simulink model "rf_satlink"  (Simulink 6.0)
settings: Solver=ode45  StartTime=0.0  StopTime=Inf  RelTol=1e-3
undefined symbols (not defined in the file or in its folder): Fs, magnitude, slcm
libraries: commrflib2 x7, commsink2 x5, dsparch4 x4, commfilt2 x2, commdigbbndam2 x2, dspsrcs4 x2, simulink x1, dspsnks4 x1, commrandsrc2 x1
CloseFcn:
  | clear satlinkSigsOut method model_type
settings Model: Creator=mclune  LastModifiedBy=arodrigu  ExtModeAutoUpdateStatusClock=off  BufferReuse=off
settings DataIOCC: SaveOutput=off  SaveTime=off  SignalLoggingName=satlinkSigsOut
settings OptimizationCC: OptimizeBlockIOStorage=off  BufferReuse=off  ExpressionFolding=off  LocalBlockOutputs=off
settings DebuggingCC: CheckExecutionContextPreStartOutputMsg=on  CheckExecutionContextRuntimeOutputMsg=on  SolverPrmCheckMsg=none  InheritedTsInSrcMsg=none
settings HardwareCC: TargetUnknown=on
settings ModelReferenceCC: UpdateModelReferenceTargets=IfOutOfDate

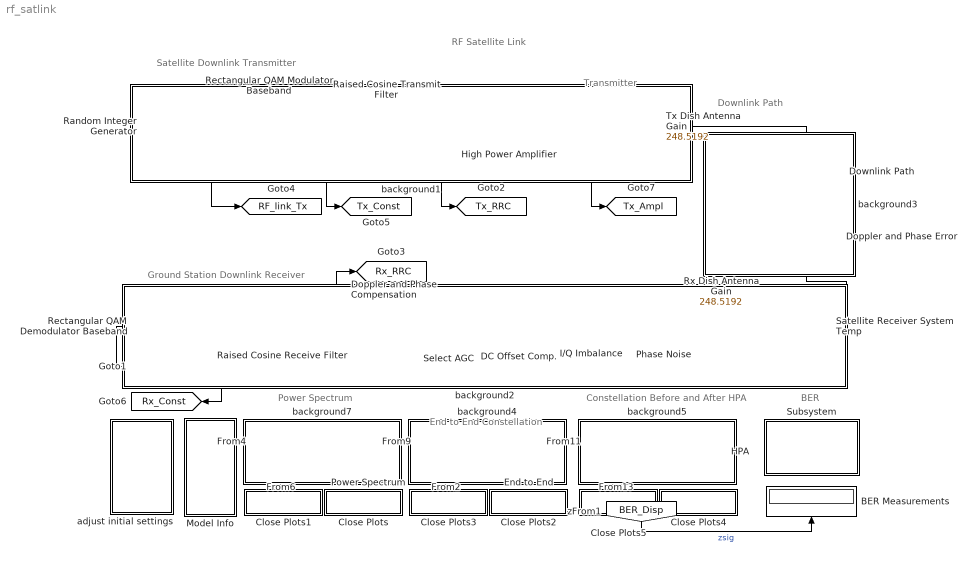
== system rf_satlink ==
  note: RF Satellite Link
  note: Constellation Before and After HPA
  note: Power Spectrum
  note: Downlink Path
  note: Satellite Downlink Transmitter
  note: Transmitter
  note: Ground Station Downlink Receiver
  note: End to End Constellation
  note: BER
  BER Measurements : Display
      settings: Orientation=up
  Close Plots : Subsystem  PropExecContextAcrossSSBoundary=on
      settings: OpenFcn=|
      | sdspfscope2([],[],[],'ScopeUpdate',[gcs '/Power Spectrum/Tx and Rx Spectrum'],'CloseFig');
      | set_param([gcs '/Power Spectrum/Tx and Rx Spectrum'],'OpenScopeAtSimStart','off');
      mask Display: disp('Close Scopes');
  Close Plots1 : Subsystem  PropExecContextAcrossSSBoundary=on
      settings: OpenFcn=|
      | sdspfscope2([],[],[],'ScopeUpdate',[gcs '/Power Spectrum/Tx and Rx Spectrum'],'OpenFig');
      | set_param([gcs '/Power Spectrum/Tx and Rx Spectrum'],'OpenScopeAtSimStart','on');
      mask Display: disp('Open Scopes');
  Close Plots2 : Subsystem  PropExecContextAcrossSSBoundary=on
      settings: OpenFcn=|
      | sdspfscope2([],[],[],'ScopeUpdate',[gcs '/End to End/Transmit Constellation'],'CloseFig');
      |    sdspfscope2([],[],[],'ScopeUpdate',[gcs '/End to End/Received Constellation'],'CloseFig');
      |  set_param([gcs '/End to End/Transmit Constellation'],'OpenScopeAtSimStart','off');
      |    set_param([gcs '/End to End/Received Constellation'],'OpenScopeAtSimStart','off');
      mask Display: disp('Close Scopes');
  Close Plots3 : Subsystem  PropExecContextAcrossSSBoundary=on
      settings: OpenFcn=|
      | sdspfscope2([],[],[],'ScopeUpdate',[gcs '/End to End/Transmit Constellation'],'OpenFig');
      |     sdspfscope2([],[],[],'ScopeUpdate',[gcs '/End to End/Received Constellation'],'OpenFig');
      |   set_param([gcs '/End to End/Transmit Constellation'],'OpenScopeAtSimStart','on');
      |     set_param([gcs '/End to End/Received Constellation'],'OpenScopeAtSimStart','on');
      mask Display: disp('Open Scopes');
  Close Plots4 : Subsystem  PropExecContextAcrossSSBoundary=on
      settings: OpenFcn=|
      | sdspfscope2([],[],[],'ScopeUpdate',[gcs '/HPA/Transmit RRC filtered signal'],'CloseFig');
      |   set_param([gcs '/HPA/Transmit RRC filtered signal'],'OpenScopeAtSimStart','off');
      |     sdspfscope2([],[],[],'ScopeUpdate',[gcs '/HPA/RRC signal after HPA'],'CloseFig');
      |   set_param([gcs '/HPA/RRC signal after HPA'],'OpenScopeAtSimStart','off');
      mask Display: disp('Close Scopes');
  Close Plots5 : Subsystem  PropExecContextAcrossSSBoundary=on
      settings: OpenFcn=|
      | sdspfscope2([],[],[],'ScopeUpdate',[gcs '/HPA/Transmit RRC filtered signal'],'OpenFig');
      | set_param([gcs '/HPA/Transmit RRC filtered signal'],'OpenScopeAtSimStart','on');
      |   sdspfscope2([],[],[],'ScopeUpdate',[gcs '/HPA/RRC signal after HPA'],'OpenFig');
      | set_param([gcs '/HPA/RRC signal after HPA'],'OpenScopeAtSimStart','on');
      mask Display: disp('Open Scopes');
  DC Offset Comp. : Subsystem  Orientation=left  BlockChoice=Magnitude Only  PropExecContextAcrossSSBoundary=on
      mask Display: disp('DC\nRemoval')
  Doppler and Phase Error : commrflib2/Phase// Frequency Offset  Orientation=down  freqOffset=0  phaseOffset=0
  Doppler and Phase Compensation : commrflib2/Phase// Frequency Offset  Orientation=left  freqOffset=0  phaseOffset=0
  Downlink Path : commrflib2/Free Space Path Loss  Orientation=down  mode=Distance and Frequency  dB=180  d=35600  fc=8000
  End to End : Subsystem  TreatAsAtomicUnit=on  PropExecContextAcrossSSBoundary=on
      mask Display: disp('End-End\nScatter\nPlot')
  HPA : Subsystem  TreatAsAtomicUnit=on  PropExecContextAcrossSSBoundary=on
      mask Display: disp('HPA\nScatter\nPlot')
  High Power Amplifier : commrflib2/Memoryless Nonlinearity  model_select=Saleh model  linGaindB=16  GindB=-21.5957  iip3=30  am2pm=1  amam=[2.1587 1.1517]  ampm=[4.0330 9.1040]  x=[8.1081 1.5413 6.5202 -0.0718]  y=[4.6645 2.0965 10.88 -0.003]  p=0.3  GoutdB=32.9118  vsat=100
  I/Q Imbalance : commrflib2/I//Q Imbalance  Orientation=left  ampImbal=0  phsImbal=0  Idc=0  Qdc=0
  Model Info : Subsystem  LoadFcn=slcm LoadBlock;  InitFcn=slcm('UpdateAllCMBlocksInThisModelInit')  PropExecContextAcrossSSBoundary=on  mask(CMBlock){InitialSaveTempField=, InitialBlockCM=None, BlockCM=None, Frame=on, SaveTempField=, DisplayStringWithTags=Info, MaskDisplayString=Info, HorizontalTextAlignment=Center, LeftAlignmentValue=0.5, SourceBlockDiagram=rf_satlink, TagMaxNumber=20, CMTag1=, CMTag2=, CMTag3=, CMTag4=, CMTag5=, CMTag6=, CMTag7=, CMTag8=, CMTag9=, CMTag10=, CMTag11=, CMTag12=, CMTag13=, CMTag14=, CMTag15=, CMTag16=, CMTag17=, CMTag18=, CMTag19=, CMTag20=}
      mask help: This block allows revision control information to be displayed within the model.
      settings: CopyFcn=slcm CopyBlock;  DeleteFcn=slcm Cancel;  PostSaveFcn=slcm('UpdateAllCMBlocksInThisModel')  NameChangeFcn=slcm Rename;  OpenFcn=commdemohelp;
      mask Display: text(str2num(LeftAlignmentValue), 0.5, MaskDisplayString, 'HorizontalAlignment', HorizontalTextAlignment)
  Phase Noise : commrflib2/Phase Noise  Orientation=left  PhNs=-100  Fo=100  seed=2137
  Power Spectrum : Subsystem  TreatAsAtomicUnit=on  PropExecContextAcrossSSBoundary=on
      mask Display: disp('Power\nSpectrum')
  Raised Cosine Receive Filter : commfilt2/Raised Cosine Receive Filter  Orientation=left  filtType=Square root  N=8  D=3  R=0.3  sampMode=Frame-based  rateMode=Downsampling  downFactor=8  downOffset=0  checkGain=Normalized  filterGain=1  checkCoeff=off  variableName=rcRxFilt  launchFVT=off
  Raised Cosine Transmit Filter : commfilt2/Raised Cosine Transmit Filter  filtType=Square root  D=3  R=0.3  sampMode=Frame-based  N=8  checkGain=Normalized  filterGain=1  checkCoeff=off  variableName=rcTxFilt  launchFVT=off
  Random Integer Generator : commrandsrc2/Random Integer Generator  mul=16  seed=37  Ts=4/100000  frameBased=on  sampPerFrame=100  orient=off
  Rectangular QAM Demodulator Baseband : commdigbbndam2/Rectangular QAM Demodulator Baseband  Orientation=left  M=16  OutType=Integer  Dec=Binary  PowType=Average Power  MinDist=2  AvgPow=1  PeakPow=1  Ph=0  numSamp=1
  Rectangular QAM Modulator Baseband : commdigbbndam2/Rectangular QAM Modulator Baseband  M=16  InType=Integer  Enc=Gray  PowType=Average Power  MinDist=2  AvgPow=1  PeakPow=1  Ph=0  numSamp=1
  Rx Dish Antenna Gain : Gain  Orientation=left  Gain=248.5192  SaturateOnIntegerOverflow=on
  Satellite Receiver System Temp : commrflib2/Receiver Thermal Noise  Orientation=left  method=Noise temperature  ntemp=0  nfigure=3.01  nfactor=2  seed=67987
  Select AGC : Subsystem  Orientation=left  AncestorBlock=rf_agc_sel/Select AGC  PropExecContextAcrossSSBoundary=on  mask{swCase=Magnitude}
      mask prompts: swCase "Case Value:"
      mask init:
      | charCase = char(swCase);
      | switch charCase,
      | case 'I and Q',
      | 		selValue = 1;
      | otherwise,
      | 		selValue = 0;
      | end
      mask StyleString: popup(Magnitude|I and Q)
      mask Display: disp([char(swCase) '\nAGC'])
  Subsystem : Subsystem  PropExecContextAcrossSSBoundary=on
      mask Display: disp('Display Complete\nBit Error Rate\nInformation');
  Tx Dish Antenna Gain : Gain  Gain=248.5192  SaturateOnIntegerOverflow=on
  adjust initial settings : Subsystem  PropExecContextAcrossSSBoundary=on  mask(RF Link Demo:Initial Settings){altitude=35600, frequency=8000, antDiam=[2 2], selTemp=0 (no noise), selLvlBO=30 dB  (negligible nonlinearity), selCorrPh=None, selDopper=None, selNoPh=Negligible (-100 dBc/Hz @ 100 Hz), selImbal=None, selDcOffset=Disabled, selAGC=Magnitude only}
      mask prompts: altitude "Satellite altitude (km):"; frequency "Frequency (MHz):"; antDiam "Transmit and receive antenna sizes (m):"; selTemp "Noise temperature (K):"; selLvlBO "HPA backoff level:"; selCorrPh "Phase correction:"; selDopper "Doppler error:"; selNoPh "Phase noise:"; selImbal "I/Q imbalance:"; selDcOffset "DC offset compensation:"; selAGC "AGC type:"
      mask help: Select the scenarios from the mask to change the link parameters. Each of the mask parameters sets the parameters in the corresponding RF impairment block(s).
      mask init:
      | eStr = rf_link_mask(gcb,'init');
      | 
      | if(isfield(eStr,'emsg') & ~isempty(eStr.emsg))
      | 	errordlg(eStr.emsg);
      | end
      | if(isfield(eStr,'emsg_w') & ~isempty(eStr.emsg_w))
      | 	warndlg(eStr.emsg_w);
      | end
      mask StyleString: edit,edit,edit,popup(0 (no noise)|20 (very low noise level)|290 (typical noise level)),popup(30 dB  (negligible nonlinearity)|7 dB  (moderate nonlinearity)|1 dB  (severe nonlinearity)),popup(None|Correct for moderate HPA AM to PM|Correct for severe HPA AM to PM),popup(None|Doppler (0.7 Hz - uncorrected)|Doppler (3 Hz - corrected)),popup(Negligible (-100 dBc/Hz @ 100 Hz)|Low  (-55 dBc/Hz @ 100 Hz)|High  (-48 dBc/Hz @ 100 Hz)),popup(None|Amplitude imbalance (3 dB)|Phase imbalance (20 deg)|In-phase DC offset (2e-6)|Quadrature DC offset (1e-5)),popup(Disabled|Enabled),popup(Magnitude only|Independent I and Q)
      mask CallbackString: rf_link_mask(gcb,'cbAltitude');|rf_link_mask(gcb,'cbFrequency');|rf_link_mask(gcb,'cbAntDiam');|rf_link_mask(gcb,'cbSelTemp');|rf_link_mask(gcb,'cbSelLvlSat');|rf_link_mask(gcb,'cbSelCorrPh');|rf_link_mask(gcb,'cbSelDopper');|rf_link_mask(gcb,'cbSelNoPh');|rf_link_mask(gcb,'cbSelImbal');|rf_link_mask(gcb,'cbDcOffset');|rf_link_mask(gcb,'cbSelAGC');
      mask Display: disp('RF Link\nDemo:\nSettings');
  background1 : Subsystem  PropExecContextAcrossSSBoundary=on
      mask Display: disp('')
  background2 : Subsystem  PropExecContextAcrossSSBoundary=on
      mask Display: disp('')
  background3 : Subsystem  PropExecContextAcrossSSBoundary=on
      mask Display: disp('')
  background4 : Subsystem  PropExecContextAcrossSSBoundary=on
      mask Display: disp('')
  background5 : Subsystem  PropExecContextAcrossSSBoundary=on
      mask Display: disp('')
  background7 : Subsystem  PropExecContextAcrossSSBoundary=on
      mask Display: disp('')
  tag scope: RF_link_Rx=global, RF_link_Tx=global, Rx_Const=global, Rx_RRC=global, Tx_Ampl=global, Tx_Const=global, Tx_RRC=global
  wires:
  Rectangular QAM Modulator Baseband/1 -> [Tx_Const], Raised Cosine Transmit Filter/1
  I/Q Imbalance/1 -> DC Offset Comp./1(In1)
  Tx Dish Antenna Gain/1 -> Downlink Path/1
  High Power Amplifier/1 -> Tx Dish Antenna Gain/1, [Tx_Ampl]
  Doppler and Phase Compensation/1 -> [Rx_RRC], Raised Cosine Receive Filter/1
  Select AGC/1(Out1) -> Doppler and Phase Compensation/1
  Satellite Receiver System Temp/1 -> Rx Dish Antenna Gain/1
  Phase Noise/1 -> I/Q Imbalance/1
  Random Integer Generator/1 -> Rectangular QAM Modulator Baseband/1, [RF_link_Tx]
  Rectangular QAM Demodulator Baseband/1 -> [RF_link_Rx]
  [Tx_RRC] -> HPA/1(In2)
  [Tx_RRC] -> Power Spectrum/1(In1)
  [Rx_RRC] -> Power Spectrum/2(In2)
  Rx Dish Antenna Gain/1 -> Phase Noise/1
  Downlink Path/1 -> Doppler and Phase Error/1
  [Rx_Const] -> End to End/2(In4)
  [Tx_Const] -> End to End/1(In1)
  [Tx_Ampl] -> HPA/2(In3)
  Doppler and Phase Error/1 -> Satellite Receiver System Temp/1
  [BER_Disp] -> BER Measurements/1  "zsig"
  DC Offset Comp./1(Out1) -> Select AGC/1(In2)
  Raised Cosine Transmit Filter/1 -> High Power Amplifier/1, [Tx_RRC]
  Raised Cosine Receive Filter/1 -> Rectangular QAM Demodulator Baseband/1, [Rx_Const]

== system rf_satlink/Close Plots ==

== system rf_satlink/Close Plots1 ==

== system rf_satlink/Close Plots2 ==

== system rf_satlink/Close Plots3 ==

== system rf_satlink/Close Plots4 ==

== system rf_satlink/Close Plots5 ==

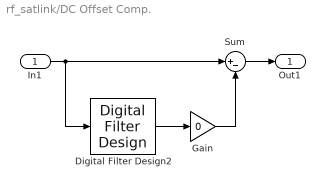
== system rf_satlink/DC Offset Comp. ==
  In1 : Inport  LatchInput=off
  Digital Filter Design2 : dsparch4/Digital Filter Design
  Gain : Gain  Gain=0  SaturateOnIntegerOverflow=on
  Sum : Sum  Inputs=|+-  SaturateOnIntegerOverflow=on
  Out1 : Outport
  wires:
  In1/1 -> Sum/1, Digital Filter Design2/1
  Gain/1 -> Sum/2
  Digital Filter Design2/1 -> Gain/1
  Sum/1 -> Out1/1

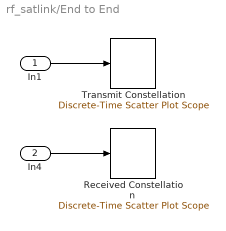
== system rf_satlink/End to End ==
  In1 : Inport  LatchInput=off
  In4 : Inport  Port=2  LatchInput=off
  Received Constellation : commsink2/Discrete-Time Scatter Plot Scope  Tag=ScatterPlot  sampPerSymb=8  offsetEye=0  numTraces=160  numNewFrames=40  LineMarkers=.  LineColors=r  fading=on  render=off  AxisGrid=on  xMin=-1.19233403062067  xMax=1.2246188834561  yMin=-1.20849372757452  yMax=1.20845918650224  inphaseLabel=In-phase Amplitude  quadratureLabel=Quadrature Amplitude  openScopeAtSimStart=on  FrameNumber=off  FigPos=[382 347 258 258]  figTitle=""  numLinesMax=50  block_type_=scatter
  Transmit Constellation : commsink2/Discrete-Time Scatter Plot Scope  Tag=ScatterPlot  sampPerSymb=8  offsetEye=0  numTraces=30  numNewFrames=30  LineMarkers=.  LineColors=b  fading=on  render=off  AxisGrid=on  xMin=-1.04355162785557  xMax=1.04829504434582  yMin=-1.04355162785557  yMax=1.04829504434582  inphaseLabel=In-phase Amplitude  quadratureLabel=Quadrature Amplitude  openScopeAtSimStart=on  FrameNumber=on  FigPos=[114 346 260 260]  figTitle=""  numLinesMax=50  block_type_=scatter
  wires:
  In1/1 -> Transmit Constellation/1
  In4/1 -> Received Constellation/1

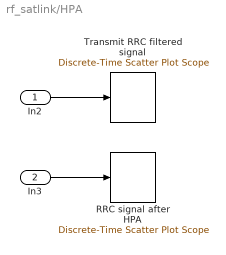
== system rf_satlink/HPA ==
  In2 : Inport  LatchInput=off
  In3 : Inport  Port=2  LatchInput=off
  RRC signal after HPA : commsink2/Discrete-Time Scatter Plot Scope  Tag=ScatterPlot  sampPerSymb=8  offsetEye=0  numTraces=200  numNewFrames=80  LineMarkers=.  LineColors=r  fading=on  render=off  AxisGrid=on  xMin=-4.02161513041803  xMax=4.01163575275656  yMin=-3.99350744429814  yMax=4.03974343887645  inphaseLabel=In-phase Amplitude  quadratureLabel=Quadrature Amplitude  openScopeAtSimStart=off  FrameNumber=off  FigPos=[422 300 243 243]  figTitle=""  numLinesMax=50  block_type_=scatter
  Transmit RRC filtered signal : commsink2/Discrete-Time Scatter Plot Scope  Tag=ScatterPlot  sampPerSymb=8  offsetEye=0  numTraces=200  numNewFrames=80  LineMarkers=.  LineColors=b  fading=on  render=off  AxisGrid=on  xMin=-0.494106248905821  xMax=0.495177369466584  yMin=-0.488837200008166  yMax=0.500446418364239  inphaseLabel=In-phase Amplitude  quadratureLabel=Quadrature Amplitude  openScopeAtSimStart=off  FrameNumber=off  FigPos=[166 310 243 243]  figTitle=""  numLinesMax=50  block_type_=scatter
  wires:
  In2/1 -> Transmit RRC filtered signal/1
  In3/1 -> RRC signal after HPA/1

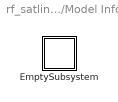
== system rf_satlink/Model Info ==
  EmptySubsystem : Subsystem  PropExecContextAcrossSSBoundary=on

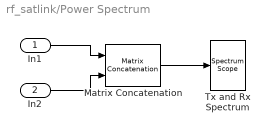
== system rf_satlink/Power Spectrum ==
  In1 : Inport  LatchInput=off
  In2 : Inport  Port=2  LatchInput=off
  Matrix Concatenation : simulink/Math Operations/Matrix Concatenation  numInports=2  catMethod=Horizontal
  Tx and Rx Spectrum : dspsnks4/Spectrum Scope  ScopeProperties=off  Domain=Frequency  HorizSpan=1  UseBuffer=on  BufferSize=512  Overlap=256  inpFftLenInherit=off  FFTlength=128  numAvg=4  DisplayProperties=on  AxisGrid=on  Memory=off  FrameNumber=off  AxisLegend=off  AxisZoom=off  OpenScopeAtSimStart=on  OpenScopeImmediately=off  FigPos=[649 346 260 261]  AxisProperties=off  XUnits=Hertz  XRange=[-Fs/2...Fs/2]  InheritXIncr=on  XIncr=1  XLabel=Samples  YUnits=dB  YLabel=Magnitude, dB  LineProperties=off  LineColors=b|r
      settings: AttributesFormatString=\n  YMin=-122.592488733173  YMax=21.004490174206
  wires:
  In1/1 -> Matrix Concatenation/1
  In2/1 -> Matrix Concatenation/2
  Matrix Concatenation/1 -> Tx and Rx Spectrum/1

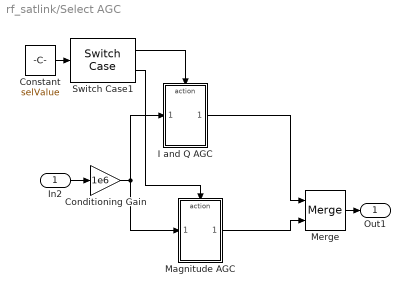
== system rf_satlink/Select AGC ==
  In2 : Inport  LatchInput=off
  Conditioning Gain : Gain  Gain=1e6  SaturateOnIntegerOverflow=on
  Constant : Constant  Value=selValue
  I and Q AGC : Subsystem  TreatAsAtomicUnit=on  PropExecContextAcrossSSBoundary=on
  Magnitude AGC : Subsystem  TreatAsAtomicUnit=on  PropExecContextAcrossSSBoundary=on
  Merge : Merge  InitialOutput=0
  Switch Case1 : SwitchCase
  Out1 : Outport
  wires:
  Switch Case1/2 -> Magnitude AGC/Action
  Switch Case1/1 -> I and Q AGC/Action
  Constant/1 -> Switch Case1/1
  In2/1 -> Conditioning Gain/1
  I and Q AGC/1(Out1) -> Merge/1
  Magnitude AGC/1(Out1) -> Merge/2
  Merge/1 -> Out1/1
  Conditioning Gain/1 -> I and Q AGC/1(In1), Magnitude AGC/1(In1)

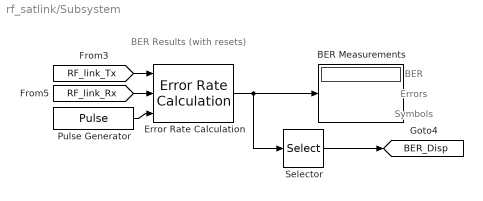
== system rf_satlink/Subsystem ==
  note: BER
  note: Errors
  note: Symbols
  note: BER Results (with resets)
  BER Measurements : Display
  Error Rate Calculation : commsink2/Error Rate Calculation  N=6  st_delay=0  cp_mode=Entire frame  subframe=[]  PMode=Port  WsName=ErrorVec  RsMode2=on  stop=off  numErr=200  maxBits=1e6
  Pulse Generator : DiscretePulseGenerator  Period=50  SampleTime=4/1000
  Selector : Selector  Elements=[1]  InputPortWidth=3
  tag scope: BER_Disp=global
  wires:
  [RF_link_Tx] -> Error Rate Calculation/1
  [RF_link_Rx] -> Error Rate Calculation/2
  Error Rate Calculation/1 -> BER Measurements/1, Selector/1
  Pulse Generator/1 -> Error Rate Calculation/3
  Selector/1 -> [BER_Disp]

== system rf_satlink/adjust initial settings ==

== system rf_satlink/background1 ==

== system rf_satlink/background2 ==

== system rf_satlink/background3 ==

== system rf_satlink/background4 ==

== system rf_satlink/background5 ==

== system rf_satlink/background7 ==

== system rf_satlink/Model Info/EmptySubsystem ==

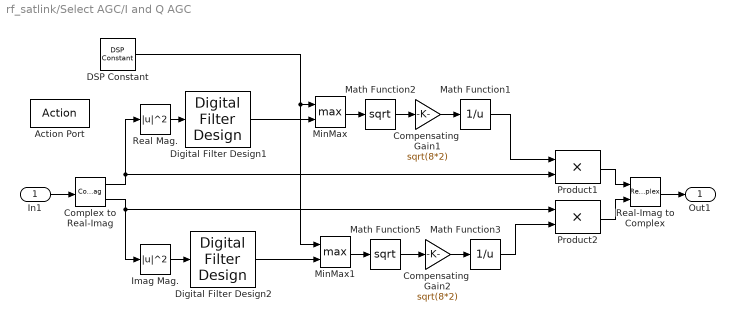
== system rf_satlink/Select AGC/I and Q AGC ==
  In1 : Inport  LatchInput=off
  Action Port : ActionPort  ActionType=case
  Compensating  Gain1 : Gain  Gain=sqrt(8*2)  SaturateOnIntegerOverflow=on
  Compensating  Gain2 : Gain  Gain=sqrt(8*2)  SaturateOnIntegerOverflow=on
  Complex to Real-Imag : ComplexToRealImag
  DSP Constant : dspsrcs4/DSP Constant  Value=eps  SampleMode=Discrete  discreteOutput=Frame-based  continuousOutput=Sample-based  sampTime=-1  framePeriod=-1  dataType=Inherit from 'Constant value'  wordLen=16  udDataType=sfix(16)  fracBitsMode=Best precision  numFracBits=15  InterpretAs1D=off  Ts=-1  FramebasedOutput=on
      settings: AttributesFormatString=\n\n\n\n
  Digital Filter Design1 : dsparch4/Digital Filter Design
  Digital Filter Design2 : dsparch4/Digital Filter Design
  Imag Mag. : Math  Operator=magnitude^2  SaturateOnIntegerOverflow=on
  Math Function1 : Math  Operator=reciprocal  SaturateOnIntegerOverflow=on
  Math Function2 : Math  Operator=sqrt  SaturateOnIntegerOverflow=on
  Math Function3 : Math  Operator=reciprocal  SaturateOnIntegerOverflow=on
  Math Function5 : Math  Operator=sqrt  SaturateOnIntegerOverflow=on
  MinMax : MinMax  Function=max  Inputs=2  SaturateOnIntegerOverflow=on  InputSameDT=on
  MinMax1 : MinMax  Function=max  Inputs=2  SaturateOnIntegerOverflow=on  InputSameDT=on
  Product1 : Product  SaturateOnIntegerOverflow=on
  Product2 : Product  SaturateOnIntegerOverflow=on
  Real Mag. : Math  Operator=magnitude^2  SaturateOnIntegerOverflow=on
  Real-Imag to Complex : RealImagToComplex
  Out1 : Outport
  wires:
  Real-Imag to Complex/1 -> Out1/1
  In1/1 -> Complex to Real-Imag/1
  Math Function3/1 -> Product2/2
  Math Function1/1 -> Product1/1
  Product2/1 -> Real-Imag to Complex/2
  Product1/1 -> Real-Imag to Complex/1
  Math Function5/1 -> Compensating  Gain2/1
  Compensating  Gain2/1 -> Math Function3/1
  Complex to Real-Imag/2 -> Product2/1, Imag Mag./1
  Complex to Real-Imag/1 -> Product1/2, Real Mag./1
  Imag Mag./1 -> Digital Filter Design2/1
  Real Mag./1 -> Digital Filter Design1/1
  Math Function2/1 -> Compensating  Gain1/1
  Compensating  Gain1/1 -> Math Function1/1
  DSP Constant/1 -> MinMax/1, MinMax1/1
  Digital Filter Design1/1 -> MinMax/2
  Digital Filter Design2/1 -> MinMax1/2
  MinMax1/1 -> Math Function5/1
  MinMax/1 -> Math Function2/1

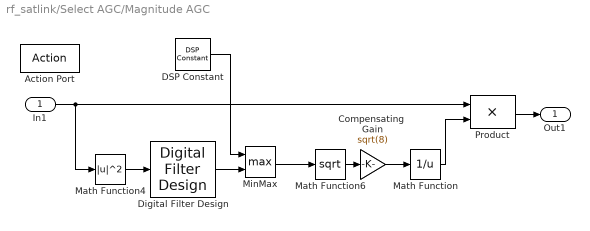
== system rf_satlink/Select AGC/Magnitude AGC ==
  In1 : Inport  LatchInput=off
  Action Port : ActionPort  ActionType=default
  Compensating  Gain : Gain  Gain=sqrt(8)  SaturateOnIntegerOverflow=on
  DSP Constant : dspsrcs4/DSP Constant  Value=eps  SampleMode=Discrete  discreteOutput=Frame-based  continuousOutput=Sample-based  sampTime=-1  framePeriod=-1  dataType=Inherit from 'Constant value'  wordLen=16  udDataType=sfix(16)  fracBitsMode=Best precision  numFracBits=15  InterpretAs1D=off  Ts=-1  FramebasedOutput=on
      settings: AttributesFormatString=\n\n\n\n
  Digital Filter Design : dsparch4/Digital Filter Design
  Math Function : Math  Operator=reciprocal  SaturateOnIntegerOverflow=on
  Math Function4 : Math  Operator=magnitude^2  SaturateOnIntegerOverflow=on
  Math Function6 : Math  Operator=sqrt  SaturateOnIntegerOverflow=on
  MinMax : MinMax  Function=max  Inputs=2  SaturateOnIntegerOverflow=on  InputSameDT=on
  Product : Product  SaturateOnIntegerOverflow=on
  Out1 : Outport
  wires:
  Product/1 -> Out1/1
  In1/1 -> Math Function4/1, Product/1
  Compensating  Gain/1 -> Math Function/1
  Math Function6/1 -> Compensating  Gain/1
  Math Function4/1 -> Digital Filter Design/1
  Math Function/1 -> Product/2
  Digital Filter Design/1 -> MinMax/2
  MinMax/1 -> Math Function6/1
  DSP Constant/1 -> MinMax/1
